simulink model "zyl73"  (R2021b)
settings: Solver=ode45  StartTime=0.0  StopTime=10  RelTol=1e-3
settings Model: Creator=zhonghuatu  LastModifiedBy=zhonghuatu

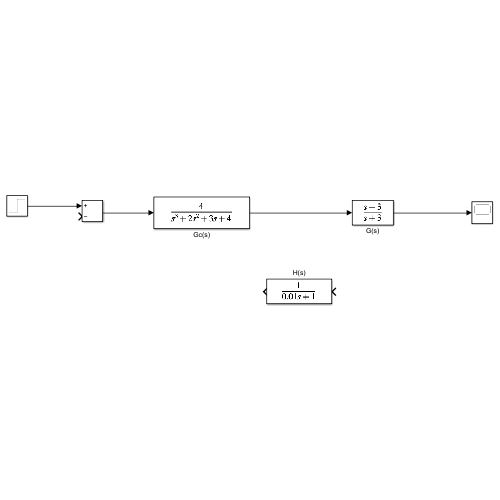
[thumbnail: Simulink's stored preview of the top-level diagram]
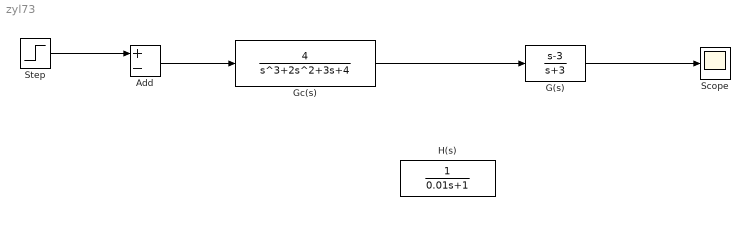
== system zyl73 ==
  Add : Sum  Inputs=+-
  G(s) : TransferFcn  Numerator=[1 -3]  Denominator=[1 3]
  Gc(s) : TransferFcn  Numerator=[4]  Denominator=[1 2 3 4]
  H(s) : TransferFcn  Denominator=[0.01 1]
  Scope : Scope
  Step : Step  SampleTime=0
  wires:
  Step/1 -> Add/1
  Add/1 -> Gc(s)/1
  Gc(s)/1 -> G(s)/1
  G(s)/1 -> Scope/1
